simulink model "TurbineModelling"  (R2016a)
settings: Solver=VariableStepAuto  StartTime=0.0  StopTime=10.0  RelTol=1e-3
libraries: powerlib x1
settings Model: Creator=ikuma  LastModifiedBy=ikuma

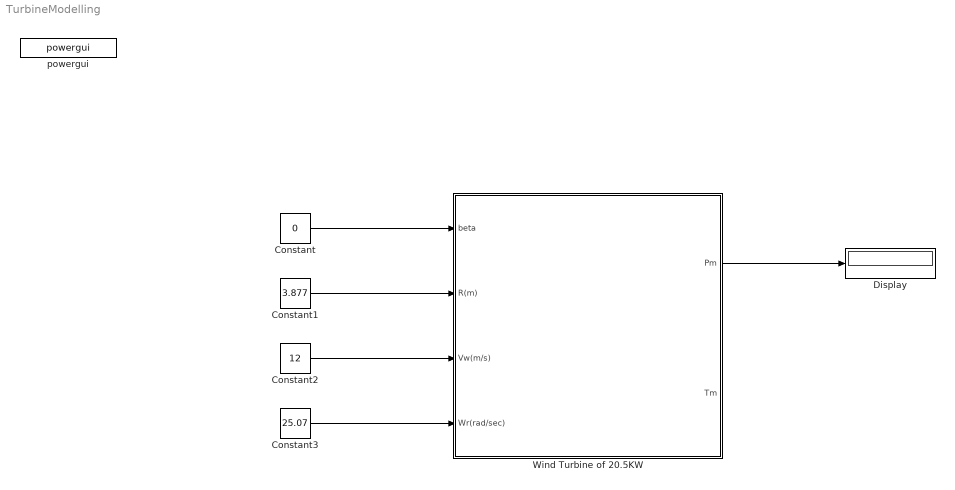
== system TurbineModelling ==
  Constant : Constant  Value=0
  Constant1 : Constant  Value=3.877
  Constant2 : Constant  Value=12
  Constant3 : Constant  Value=25.07
  Display : Display
      settings: Format=bank
  Wind Turbine of 20.5KW : Subsystem
  powergui : powerlib/powergui  Priority=1  SimulationMode=Continuous  SolverType=Tustin/Backward Euler (TBE)  SampleTime=50e-6  frequency=60  SPID=off  DisableSnubberDevices=off  DisableRonSwitches=off  DisableVfSwitches=off  SwTol=0  DisplayEquations=off  Interpol=off  ExternalGateDelay=off  methode=off  Ts=10  FunctionMessages=off  echomessages=off  HookPort=off  EnableUseOfTLC=off  x0status=blocks  frequencyindice=60  Pbase=100e6  ErrMax=1e-4  Iterations=50  UnitsV=kV  UnitsW=MW  buscounter=0  RestoreLinks=warning  ResistiveCurrentMeasurement=off  Frange=[0:2:500]  Ylog=off  Xlog=on  ShowGrid=off  save=off  variable=ZData  structure=0  ZoomFFT=off  StartTime=0.0  cycles=1  DisplayStyle=1  fundamental=60  FreqAxis=off  MaxFrequency=1000  frequencyindicesteady=1  RmsSteady=1  display=off
  wires:
  Constant3/1 -> Wind Turbine of 20.5KW/4(Wr(rad/sec))
  Constant2/1 -> Wind Turbine of 20.5KW/3(Vw(m/s))
  Constant1/1 -> Wind Turbine of 20.5KW/2(R(m))
  Constant/1 -> Wind Turbine of 20.5KW/1(beta)
  Wind Turbine of 20.5KW/1(Pm) -> Display/1

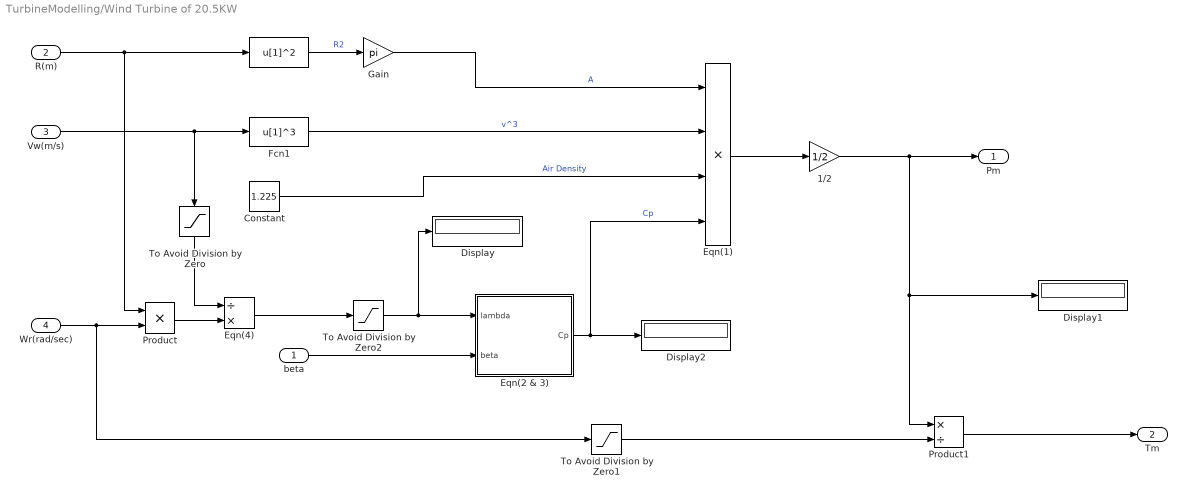
== system TurbineModelling/Wind Turbine of 20.5KW ==
  beta : Inport
  R(m) : Inport  Port=2
  Vw(m/s) : Inport  Port=3
  Wr(rad/sec) : Inport  Port=4
  " " : Fcn  Expr=u[1]^2
  1/2 : Gain  Gain=1/2
  Constant : Constant  Value=1.225
  Display : Display
  Display1 : Display
      settings: Format=bank
  Display2 : Display
  Eqn(1) : Product  Inputs=****
  Eqn(2 & 3) : Subsystem
  Eqn(4) : Product  Inputs=/*
  Fcn1 : Fcn  Expr=u[1]^3
  Gain : Gain  Gain=pi
  Product : Product
  Product1 : Product  Inputs=*/
  To Avoid Division by Zero : Saturate  UpperLimit=1e6  LowerLimit=1e-6
  To Avoid Division by Zero1 : Saturate  UpperLimit=1e6  LowerLimit=1e-6
  To Avoid Division by Zero2 : Saturate  UpperLimit=inf  LowerLimit=1e-6
  Pm : Outport
  Tm : Outport  Port=2
  wires:
  1/2/1 -> Display1/1, Product1/1, Pm/1
  Eqn(1)/1 -> 1/2/1
  Eqn(2 & 3)/1(Cp) -> Display2/1, Eqn(1)/4  "Cp"
  Constant/1 -> Eqn(1)/3  "Air Density"
  Fcn1/1 -> Eqn(1)/2  "v^3"
  Gain/1 -> Eqn(1)/1  "A"
  R(m)/1 -> Product/1, " "/1
  " "/1 -> Gain/1  "R2"
  Vw(m/s)/1 -> Fcn1/1, To Avoid Division by Zero/1
  Wr(rad/sec)/1 -> To Avoid Division by Zero1/1, Product/2
  Product/1 -> Eqn(4)/2
  Eqn(4)/1 -> To Avoid Division by Zero2/1
  To Avoid Division by Zero/1 -> Eqn(4)/1
  beta/1 -> Eqn(2 & 3)/2(beta)
  Product1/1 -> Tm/1
  To Avoid Division by Zero1/1 -> Product1/2
  To Avoid Division by Zero2/1 -> Display/1, Eqn(2 & 3)/1(lambda)

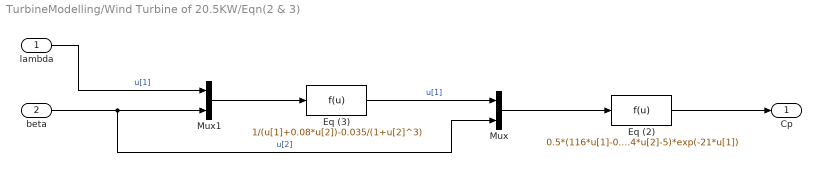
== system TurbineModelling/Wind Turbine of 20.5KW/Eqn(2 & 3) ==
  lambda : Inport
  beta : Inport  Port=2
  "Eq (2) " : Fcn  Expr=0.5*(116*u[1]-0.4*u[2]-5)*exp(-21*u[1])
  Eq (3) : Fcn  Expr=1/(u[1]+0.08*u[2])-0.035/(1+u[2]^3)
  Mux : Mux  Inputs=2
  Mux1 : Mux  Inputs=2
  Cp : Outport
  wires:
  "Eq (2) "/1 -> Cp/1
  Mux/1 -> "Eq (2) "/1
  Eq (3)/1 -> Mux/1  "u[1]"
  beta/1 -> Mux/2, Mux1/2  "u[2]"
  lambda/1 -> Mux1/1  "u[1]"
  Mux1/1 -> Eq (3)/1
